simulink library "AEMS_Standard_Library"  (R2016b)
settings: Solver=ode45  StartTime=0.0  StopTime=10.0  RelTol=1e-3
undefined symbols (not defined in the file or in its folder): BkPY, carto, Cbx_extegr, Cbx_lpegrsys, Cbx_portegr, Cnx_bnk_nr_conf, Cnx_cyl_nr_conf, ConfigManagement, configuration_management, Cxx_dcm_io_tmr_end_xxxx, Cxx_dcm_rt_tmr_end, Cxx_DID_xxxx_IO_max, Cxx_DID_xxxx_IO_min, Cxx_egrhsofs, Cxx_vmaniegi, DEM_DEBOUNCE_FREEZE, DEM_DTR_CTL_INVISIBLE, DEM_DTR_CTL_NORMAL, Dem_DtrId2_XXX, Dem_DtrId3_XXX, Dem_DtrId4_XXX, Dem_DtrId5_XXX, Dem_DtrId6_XXX, Dem_DtrId7_XXX, Dem_DtrId8_XXX, Dem_DtrId9_XXX, Dem_DtrId_XXX, Dem_EnableConditionId2_XXX, Dem_EnableConditionId3_XXX, Dem_EnableConditionId4_XXX, Dem_EnableConditionId5_XXX, Dem_EnableConditionId6_XXX, Dem_EnableConditionId7_XXX, Dem_EnableConditionId8_XXX, Dem_EnableConditionId_XXX, Dem_EventId, Dem_EventId2_XXX, Dem_EventId3_XXX, Dem_EventId4_XXX, Dem_EventId5_XXX, Dem_EventId6_XXX, Dem_EventId7_XXX, Dem_EventId8_XXX, Dem_EventId9_XXX, Dem_EventId_Device_Faulttype, Dem_EventId_XXX, DEM_IUMPR_GENERAL_DENOMINATOR, DEM_OPCYC_IGNITION, Dem_RatioId2_XXX, Dem_RatioId3_XXX, Dem_RatioId4_XXX, Dem_RatioId5_XXX, Dem_RatioId6_XXX, Dem_RatioId7_XXX, Dem_RatioId8_XXX, Dem_RatioId_XXX, Dem_StorageConditionId2_XXX, Dem_StorageConditionId3_XXX, Dem_StorageConditionId4_XXX, Dem_StorageConditionId5_XXX ... (+65)
libraries: AEMS_Standard_Library x477, simulink x2
(part 33 of 39)

== system AEMS_Standard_Library/SUB/AEMS_DEM_SET_DTR_8DU/Dem_SetDTR_Call8 ==
  testresult8 : Inport  Interpolate=off
  lowerlimit8 : Inport  Port=2  Interpolate=off
  upperlimit8 : Inport  Port=3  Interpolate=off
  ctrl_flag8 : Inport  Port=4  Interpolate=off
  set_flag8 : EnablePort
      settings: AttributesFormatString=<states=%<StatesWhenEnabling>>
  AEMS_DEM_SETDTR8 : AEMS_Standard_Library/SUB/AEMS_DEM_SETDTR  Tag=[LIB]
      settings: AttributesFormatString=%<MaskType>
  Ctrlval_block1 : Constant  Value=DEM_DTR_CTL_NORMAL  OutDataTypeStr=uint8
  Ctrlval_block2 : Constant  Value=DEM_DTR_CTL_INVISIBLE  OutDataTypeStr=uint8
  DTRId_block8 : Constant  Value=Dem_DtrId8_XXX  OutDataTypeStr=uint16
  Data Type Conversion : DataTypeConversion  OutDataTypeStr=int32  SaturateOnIntegerOverflow=on
  Data Type Conversion1 : DataTypeConversion  OutDataTypeStr=int32  SaturateOnIntegerOverflow=on
  Data Type Conversion2 : DataTypeConversion  OutDataTypeStr=int32  SaturateOnIntegerOverflow=on
  Limitter22 : Saturate  UpperLimit=1  LowerLimit=0
      settings: AttributesFormatString=<limits=%<UpperLimit>/%<LowerLimit>>
  Limitter23 : Saturate  UpperLimit=1  LowerLimit=0
      settings: AttributesFormatString=<limits=%<UpperLimit>/%<LowerLimit>>
  Limitter24 : Saturate  UpperLimit=1  LowerLimit=0
      settings: AttributesFormatString=<limits=%<UpperLimit>/%<LowerLimit>>
  Sum : Sum  OutDataTypeStr=Inherit: Inherit via back propagation  SaturateOnIntegerOverflow=on  InputSameDT=on
  Sum1 : Sum  OutDataTypeStr=Inherit: Inherit via back propagation  SaturateOnIntegerOverflow=on  InputSameDT=on
  Sum2 : Sum  OutDataTypeStr=Inherit: Inherit via back propagation  SaturateOnIntegerOverflow=on  InputSameDT=on
  Switch : Switch  Criteria=u2 ~= 0  ZeroCross=off  InputSameDT=on
      settings: AttributesFormatString=Criteria=%<Criteria>
  offset1 : Constant  Value=0  OutDataTypeStr=uint16
  offset2 : Constant  Value=0  OutDataTypeStr=uint16
  offset3 : Constant  Value=0  OutDataTypeStr=uint16
  wires:
  Data Type Conversion2/1 -> AEMS_DEM_SETDTR8/4  "uplimit8"
  Data Type Conversion1/1 -> AEMS_DEM_SETDTR8/3  "lowlimit8"
  Data Type Conversion/1 -> AEMS_DEM_SETDTR8/2  "result8"
  DTRId_block8/1 -> AEMS_DEM_SETDTR8/1  "dtrid8"
  upperlimit8/1 -> Limitter24/1
  lowerlimit8/1 -> Limitter23/1
  testresult8/1 -> Limitter22/1
  Sum2/1 -> Data Type Conversion2/1
  Sum1/1 -> Data Type Conversion1/1
  Sum/1 -> Data Type Conversion/1
  Limitter24/1 -> Sum2/2
  offset3/1 -> Sum2/1
  Limitter23/1 -> Sum1/2
  offset2/1 -> Sum1/1
  Limitter22/1 -> Sum/2
  offset1/1 -> Sum/1
  Ctrlval_block1/1 -> Switch/1
  ctrl_flag8/1 -> Switch/2
  Ctrlval_block2/1 -> Switch/3
  Switch/1 -> AEMS_DEM_SETDTR8/5  "ctrlval8"

== system AEMS_Standard_Library/SUB/AEMS_DEM_SET_DTR_9DU/Dem_SetDTR_Call0 ==
  testresult0 : Inport  Interpolate=off
      settings: AttributesFormatString=<tsample=%<SampleTime>>
  lowerlimit0 : Inport  Port=2  Interpolate=off
      settings: AttributesFormatString=<tsample=%<SampleTime>>
  upperlimit0 : Inport  Port=3  Interpolate=off
      settings: AttributesFormatString=<tsample=%<SampleTime>>
  ctrl_flag0 : Inport  Port=4  Interpolate=off
      settings: AttributesFormatString=<tsample=%<SampleTime>>
  set_flag0 : EnablePort
      settings: AttributesFormatString=<states=%<StatesWhenEnabling>>
  AEMS_DEM_SETDTR : AEMS_Standard_Library/SUB/AEMS_DEM_SETDTR  Tag=[LIB]
      settings: AttributesFormatString=%<MaskType>
  Ctrlval_block1 : Constant  Value=DEM_DTR_CTL_NORMAL  OutDataTypeStr=uint8
  Ctrlval_block2 : Constant  Value=DEM_DTR_CTL_INVISIBLE  OutDataTypeStr=uint8
  DTRId_block0 : Constant  Value=Dem_DtrId_XXX  OutDataTypeStr=uint16
  Data Type Conversion : DataTypeConversion  OutDataTypeStr=int32  SaturateOnIntegerOverflow=on
  Data Type Conversion1 : DataTypeConversion  OutDataTypeStr=int32  SaturateOnIntegerOverflow=on
  Data Type Conversion2 : DataTypeConversion  OutDataTypeStr=int32  SaturateOnIntegerOverflow=on
  Limitter25 : Saturate  UpperLimit=1  LowerLimit=0
      settings: AttributesFormatString=<limits=%<UpperLimit>/%<LowerLimit>>
  Limitter26 : Saturate  UpperLimit=1  LowerLimit=0
      settings: AttributesFormatString=<limits=%<UpperLimit>/%<LowerLimit>>
  Limitter27 : Saturate  UpperLimit=1  LowerLimit=0
      settings: AttributesFormatString=<limits=%<UpperLimit>/%<LowerLimit>>
  Sum : Sum  SaturateOnIntegerOverflow=on  InputSameDT=on
  Sum1 : Sum  SaturateOnIntegerOverflow=on  InputSameDT=on
  Sum2 : Sum  SaturateOnIntegerOverflow=on  InputSameDT=on
  Switch : Switch  Threshold=0.5  ZeroCross=off  InputSameDT=on
  offset25 : Constant  Value=0  OutDataTypeStr=uint16
  offset26 : Constant  Value=0  OutDataTypeStr=uint16
  offset27 : Constant  Value=0  OutDataTypeStr=uint16
  wires:
  Ctrlval_block2/1 -> Switch/3
  ctrl_flag0/1 -> Switch/2
  Ctrlval_block1/1 -> Switch/1
  Switch/1 -> AEMS_DEM_SETDTR/5  "ctrlval0"
  offset25/1 -> Sum/1
  Limitter25/1 -> Sum/2
  offset26/1 -> Sum1/1
  Limitter26/1 -> Sum1/2
  offset27/1 -> Sum2/1
  Limitter27/1 -> Sum2/2
  Sum/1 -> Data Type Conversion/1
  Sum1/1 -> Data Type Conversion1/1
  Sum2/1 -> Data Type Conversion2/1
  testresult0/1 -> Limitter25/1
  lowerlimit0/1 -> Limitter26/1
  upperlimit0/1 -> Limitter27/1
  DTRId_block0/1 -> AEMS_DEM_SETDTR/1  "dtrid0"
  Data Type Conversion/1 -> AEMS_DEM_SETDTR/2  "result0"
  Data Type Conversion1/1 -> AEMS_DEM_SETDTR/3  "lowlimit0"
  Data Type Conversion2/1 -> AEMS_DEM_SETDTR/4  "uplimit0"

== system AEMS_Standard_Library/SUB/AEMS_DEM_SET_DTR_9DU/Dem_SetDTR_Call1 ==
  testresult1 : Inport  Interpolate=off
      settings: AttributesFormatString=<tsample=%<SampleTime>>
  lowerlimit1 : Inport  Port=2  Interpolate=off
      settings: AttributesFormatString=<tsample=%<SampleTime>>
  upperlimit1 : Inport  Port=3  Interpolate=off
      settings: AttributesFormatString=<tsample=%<SampleTime>>
  ctrl_flag1 : Inport  Port=4  Interpolate=off
      settings: AttributesFormatString=<tsample=%<SampleTime>>
  set_flag1 : EnablePort
      settings: AttributesFormatString=<states=%<StatesWhenEnabling>>
  AEMS_DEM_SETDTR : AEMS_Standard_Library/SUB/AEMS_DEM_SETDTR  Tag=[LIB]
      settings: AttributesFormatString=%<MaskType>
  Ctrlval_block1 : Constant  Value=DEM_DTR_CTL_NORMAL  OutDataTypeStr=uint8
  Ctrlval_block2 : Constant  Value=DEM_DTR_CTL_INVISIBLE  OutDataTypeStr=uint8
  DTRId_block1 : Constant  Value=Dem_DtrId2_XXX  OutDataTypeStr=uint16
  Data Type Conversion : DataTypeConversion  OutDataTypeStr=int32  SaturateOnIntegerOverflow=on
  Data Type Conversion1 : DataTypeConversion  OutDataTypeStr=int32  SaturateOnIntegerOverflow=on
  Data Type Conversion2 : DataTypeConversion  OutDataTypeStr=int32  SaturateOnIntegerOverflow=on
  Limitter1 : Saturate  UpperLimit=1  LowerLimit=0
      settings: AttributesFormatString=<limits=%<UpperLimit>/%<LowerLimit>>
  Limitter2 : Saturate  UpperLimit=1  LowerLimit=0
      settings: AttributesFormatString=<limits=%<UpperLimit>/%<LowerLimit>>
  Limitter3 : Saturate  UpperLimit=1  LowerLimit=0
      settings: AttributesFormatString=<limits=%<UpperLimit>/%<LowerLimit>>
  Sum : Sum  SaturateOnIntegerOverflow=on  InputSameDT=on
  Sum1 : Sum  SaturateOnIntegerOverflow=on  InputSameDT=on
  Sum2 : Sum  SaturateOnIntegerOverflow=on  InputSameDT=on
  Switch : Switch  Threshold=0.5  ZeroCross=off  InputSameDT=on
  offset1 : Constant  Value=0  OutDataTypeStr=uint16
  offset2 : Constant  Value=0  OutDataTypeStr=uint16
  offset3 : Constant  Value=0  OutDataTypeStr=uint16
  wires:
  Data Type Conversion2/1 -> AEMS_DEM_SETDTR/4  "uplimit1"
  Data Type Conversion1/1 -> AEMS_DEM_SETDTR/3  "lowlimit1"
  Data Type Conversion/1 -> AEMS_DEM_SETDTR/2  "result1"
  DTRId_block1/1 -> AEMS_DEM_SETDTR/1  "dtrid1"
  upperlimit1/1 -> Limitter3/1
  lowerlimit1/1 -> Limitter2/1
  testresult1/1 -> Limitter1/1
  Sum2/1 -> Data Type Conversion2/1
  Sum1/1 -> Data Type Conversion1/1
  Sum/1 -> Data Type Conversion/1
  Limitter3/1 -> Sum2/2
  offset3/1 -> Sum2/1
  Limitter2/1 -> Sum1/2
  offset2/1 -> Sum1/1
  Limitter1/1 -> Sum/2
  offset1/1 -> Sum/1
  Switch/1 -> AEMS_DEM_SETDTR/5  "ctrlval1"
  Ctrlval_block1/1 -> Switch/1
  ctrl_flag1/1 -> Switch/2
  Ctrlval_block2/1 -> Switch/3

== system AEMS_Standard_Library/SUB/AEMS_DEM_SET_DTR_9DU/Dem_SetDTR_Call2 ==
  testresult2 : Inport  Interpolate=off
      settings: AttributesFormatString=<tsample=%<SampleTime>>
  lowerlimit2 : Inport  Port=2  Interpolate=off
      settings: AttributesFormatString=<tsample=%<SampleTime>>
  upperlimit2 : Inport  Port=3  Interpolate=off
      settings: AttributesFormatString=<tsample=%<SampleTime>>
  ctrl_flag2 : Inport  Port=4  Interpolate=off
      settings: AttributesFormatString=<tsample=%<SampleTime>>
  set_flag2 : EnablePort
      settings: AttributesFormatString=<states=%<StatesWhenEnabling>>
  AEMS_DEM_SETDTR : AEMS_Standard_Library/SUB/AEMS_DEM_SETDTR  Tag=[LIB]
      settings: AttributesFormatString=%<MaskType>
  Ctrlval_block1 : Constant  Value=DEM_DTR_CTL_NORMAL  OutDataTypeStr=uint8
  Ctrlval_block2 : Constant  Value=DEM_DTR_CTL_INVISIBLE  OutDataTypeStr=uint8
  DTRId_block2 : Constant  Value=Dem_DtrId3_XXX  OutDataTypeStr=uint16
  Data Type Conversion : DataTypeConversion  OutDataTypeStr=int32  SaturateOnIntegerOverflow=on
  Data Type Conversion1 : DataTypeConversion  OutDataTypeStr=int32  SaturateOnIntegerOverflow=on
  Data Type Conversion2 : DataTypeConversion  OutDataTypeStr=int32  SaturateOnIntegerOverflow=on
  Limitter4 : Saturate  UpperLimit=1  LowerLimit=0
      settings: AttributesFormatString=<limits=%<UpperLimit>/%<LowerLimit>>
  Limitter5 : Saturate  UpperLimit=1  LowerLimit=0
      settings: AttributesFormatString=<limits=%<UpperLimit>/%<LowerLimit>>
  Limitter6 : Saturate  UpperLimit=1  LowerLimit=0
      settings: AttributesFormatString=<limits=%<UpperLimit>/%<LowerLimit>>
  Sum : Sum  SaturateOnIntegerOverflow=on  InputSameDT=on
  Sum1 : Sum  SaturateOnIntegerOverflow=on  InputSameDT=on
  Sum2 : Sum  SaturateOnIntegerOverflow=on  InputSameDT=on
  Switch : Switch  Threshold=0.5  ZeroCross=off  InputSameDT=on
  offset1 : Constant  Value=0  OutDataTypeStr=uint16
  offset2 : Constant  Value=0  OutDataTypeStr=uint16
  offset3 : Constant  Value=0  OutDataTypeStr=uint16
  wires:
  Data Type Conversion2/1 -> AEMS_DEM_SETDTR/4  "uplimit2"
  Data Type Conversion1/1 -> AEMS_DEM_SETDTR/3  "lowlimit2"
  Data Type Conversion/1 -> AEMS_DEM_SETDTR/2  "result2"
  DTRId_block2/1 -> AEMS_DEM_SETDTR/1  "dtrid2"
  upperlimit2/1 -> Limitter6/1
  lowerlimit2/1 -> Limitter5/1
  testresult2/1 -> Limitter4/1
  Sum2/1 -> Data Type Conversion2/1
  Sum1/1 -> Data Type Conversion1/1
  Sum/1 -> Data Type Conversion/1
  Limitter6/1 -> Sum2/2
  offset3/1 -> Sum2/1
  Limitter5/1 -> Sum1/2
  offset2/1 -> Sum1/1
  Limitter4/1 -> Sum/2
  offset1/1 -> Sum/1
  Ctrlval_block1/1 -> Switch/1
  ctrl_flag2/1 -> Switch/2
  Ctrlval_block2/1 -> Switch/3
  Switch/1 -> AEMS_DEM_SETDTR/5  "ctrlval2"

== system AEMS_Standard_Library/SUB/AEMS_DEM_SET_DTR_9DU/Dem_SetDTR_Call3 ==
  testresult3 : Inport  Interpolate=off
      settings: AttributesFormatString=<tsample=%<SampleTime>>
  lowerlimit3 : Inport  Port=2  Interpolate=off
      settings: AttributesFormatString=<tsample=%<SampleTime>>
  upperlimit3 : Inport  Port=3  Interpolate=off
      settings: AttributesFormatString=<tsample=%<SampleTime>>
  ctrl_flag3 : Inport  Port=4  Interpolate=off
      settings: AttributesFormatString=<tsample=%<SampleTime>>
  set_flag3 : EnablePort
      settings: AttributesFormatString=<states=%<StatesWhenEnabling>>
  AEMS_DEM_SETDTR : AEMS_Standard_Library/SUB/AEMS_DEM_SETDTR  Tag=[LIB]
      settings: AttributesFormatString=%<MaskType>
  Ctrlval_block1 : Constant  Value=DEM_DTR_CTL_NORMAL  OutDataTypeStr=uint8
  Ctrlval_block2 : Constant  Value=DEM_DTR_CTL_INVISIBLE  OutDataTypeStr=uint8
  DTRId_block3 : Constant  Value=Dem_DtrId4_XXX  OutDataTypeStr=uint16
  Data Type Conversion : DataTypeConversion  OutDataTypeStr=int32  SaturateOnIntegerOverflow=on
  Data Type Conversion1 : DataTypeConversion  OutDataTypeStr=int32  SaturateOnIntegerOverflow=on
  Data Type Conversion2 : DataTypeConversion  OutDataTypeStr=int32  SaturateOnIntegerOverflow=on
  Limitter7 : Saturate  UpperLimit=1  LowerLimit=0
      settings: AttributesFormatString=<limits=%<UpperLimit>/%<LowerLimit>>
  Limitter8 : Saturate  UpperLimit=1  LowerLimit=0
      settings: AttributesFormatString=<limits=%<UpperLimit>/%<LowerLimit>>
  Limitter9 : Saturate  UpperLimit=1  LowerLimit=0
      settings: AttributesFormatString=<limits=%<UpperLimit>/%<LowerLimit>>
  Sum : Sum  SaturateOnIntegerOverflow=on  InputSameDT=on
  Sum1 : Sum  SaturateOnIntegerOverflow=on  InputSameDT=on
  Sum2 : Sum  SaturateOnIntegerOverflow=on  InputSameDT=on
  Switch : Switch  Threshold=0.5  ZeroCross=off  InputSameDT=on
  offset1 : Constant  Value=0  OutDataTypeStr=uint16
  offset2 : Constant  Value=0  OutDataTypeStr=uint16
  offset3 : Constant  Value=0  OutDataTypeStr=uint16
  wires:
  Data Type Conversion2/1 -> AEMS_DEM_SETDTR/4  "uplimit3"
  Data Type Conversion1/1 -> AEMS_DEM_SETDTR/3  "lowlimit3"
  Data Type Conversion/1 -> AEMS_DEM_SETDTR/2  "result3"
  DTRId_block3/1 -> AEMS_DEM_SETDTR/1  "dtrid3"
  upperlimit3/1 -> Limitter9/1
  lowerlimit3/1 -> Limitter8/1
  testresult3/1 -> Limitter7/1
  Sum2/1 -> Data Type Conversion2/1
  Sum1/1 -> Data Type Conversion1/1
  Sum/1 -> Data Type Conversion/1
  Limitter9/1 -> Sum2/2
  offset3/1 -> Sum2/1
  Limitter8/1 -> Sum1/2
  offset2/1 -> Sum1/1
  Limitter7/1 -> Sum/2
  offset1/1 -> Sum/1
  Ctrlval_block1/1 -> Switch/1
  ctrl_flag3/1 -> Switch/2
  Ctrlval_block2/1 -> Switch/3
  Switch/1 -> AEMS_DEM_SETDTR/5  "ctrlval3"

== system AEMS_Standard_Library/SUB/AEMS_DEM_SET_DTR_9DU/Dem_SetDTR_Call4 ==
  testresult4 : Inport  Interpolate=off
      settings: AttributesFormatString=<tsample=%<SampleTime>>
  lowerlimit4 : Inport  Port=2  Interpolate=off
      settings: AttributesFormatString=<tsample=%<SampleTime>>
  upperlimit4 : Inport  Port=3  Interpolate=off
      settings: AttributesFormatString=<tsample=%<SampleTime>>
  ctrl_flag4 : Inport  Port=4  Interpolate=off
      settings: AttributesFormatString=<tsample=%<SampleTime>>
  set_flag4 : EnablePort
      settings: AttributesFormatString=<states=%<StatesWhenEnabling>>
  AEMS_DEM_SETDTR : AEMS_Standard_Library/SUB/AEMS_DEM_SETDTR  Tag=[LIB]
      settings: AttributesFormatString=%<MaskType>
  Ctrlval_block1 : Constant  Value=DEM_DTR_CTL_NORMAL  OutDataTypeStr=uint8
  Ctrlval_block2 : Constant  Value=DEM_DTR_CTL_INVISIBLE  OutDataTypeStr=uint8
  DTRId_block4 : Constant  Value=Dem_DtrId5_XXX  OutDataTypeStr=uint16
  Data Type Conversion : DataTypeConversion  OutDataTypeStr=int32  SaturateOnIntegerOverflow=on
  Data Type Conversion1 : DataTypeConversion  OutDataTypeStr=int32  SaturateOnIntegerOverflow=on
  Data Type Conversion2 : DataTypeConversion  OutDataTypeStr=int32  SaturateOnIntegerOverflow=on
  Limitter10 : Saturate  UpperLimit=1  LowerLimit=0
      settings: AttributesFormatString=<limits=%<UpperLimit>/%<LowerLimit>>
  Limitter11 : Saturate  UpperLimit=1  LowerLimit=0
      settings: AttributesFormatString=<limits=%<UpperLimit>/%<LowerLimit>>
  Limitter12 : Saturate  UpperLimit=1  LowerLimit=0
      settings: AttributesFormatString=<limits=%<UpperLimit>/%<LowerLimit>>
  Sum : Sum  SaturateOnIntegerOverflow=on  InputSameDT=on
  Sum1 : Sum  SaturateOnIntegerOverflow=on  InputSameDT=on
  Sum2 : Sum  SaturateOnIntegerOverflow=on  InputSameDT=on
  Switch : Switch  Threshold=0.5  ZeroCross=off  InputSameDT=on
  offset1 : Constant  Value=0  OutDataTypeStr=uint16
  offset2 : Constant  Value=0  OutDataTypeStr=uint16
  offset3 : Constant  Value=0  OutDataTypeStr=uint16
  wires:
  Data Type Conversion2/1 -> AEMS_DEM_SETDTR/4  "uplimit4"
  Data Type Conversion1/1 -> AEMS_DEM_SETDTR/3  "lowlimit4"
  Data Type Conversion/1 -> AEMS_DEM_SETDTR/2  "result4"
  DTRId_block4/1 -> AEMS_DEM_SETDTR/1  "dtrid4"
  upperlimit4/1 -> Limitter12/1
  lowerlimit4/1 -> Limitter11/1
  testresult4/1 -> Limitter10/1
  Sum2/1 -> Data Type Conversion2/1
  Sum1/1 -> Data Type Conversion1/1
  Sum/1 -> Data Type Conversion/1
  Limitter12/1 -> Sum2/2
  offset3/1 -> Sum2/1
  Limitter11/1 -> Sum1/2
  offset2/1 -> Sum1/1
  Limitter10/1 -> Sum/2
  offset1/1 -> Sum/1
  Ctrlval_block1/1 -> Switch/1
  ctrl_flag4/1 -> Switch/2
  Ctrlval_block2/1 -> Switch/3
  Switch/1 -> AEMS_DEM_SETDTR/5  "ctrlval4"

== system AEMS_Standard_Library/SUB/AEMS_DEM_SET_DTR_9DU/Dem_SetDTR_Call5 ==
  testresult5 : Inport  Interpolate=off
      settings: AttributesFormatString=<tsample=%<SampleTime>>
  lowerlimit5 : Inport  Port=2  Interpolate=off
      settings: AttributesFormatString=<tsample=%<SampleTime>>
  upperlimit5 : Inport  Port=3  Interpolate=off
      settings: AttributesFormatString=<tsample=%<SampleTime>>
  ctrl_flag5 : Inport  Port=4  Interpolate=off
      settings: AttributesFormatString=<tsample=%<SampleTime>>
  set_flag5 : EnablePort
      settings: AttributesFormatString=<states=%<StatesWhenEnabling>>
  AEMS_DEM_SETDTR : AEMS_Standard_Library/SUB/AEMS_DEM_SETDTR  Tag=[LIB]
      settings: AttributesFormatString=%<MaskType>
  Ctrlval_block1 : Constant  Value=DEM_DTR_CTL_NORMAL  OutDataTypeStr=uint8
  Ctrlval_block2 : Constant  Value=DEM_DTR_CTL_INVISIBLE  OutDataTypeStr=uint8
  DTRId_block5 : Constant  Value=Dem_DtrId6_XXX  OutDataTypeStr=uint16
  Data Type Conversion : DataTypeConversion  OutDataTypeStr=int32  SaturateOnIntegerOverflow=on
  Data Type Conversion1 : DataTypeConversion  OutDataTypeStr=int32  SaturateOnIntegerOverflow=on
  Data Type Conversion2 : DataTypeConversion  OutDataTypeStr=int32  SaturateOnIntegerOverflow=on
  Limitter13 : Saturate  UpperLimit=1  LowerLimit=0
      settings: AttributesFormatString=<limits=%<UpperLimit>/%<LowerLimit>>
  Limitter14 : Saturate  UpperLimit=1  LowerLimit=0
      settings: AttributesFormatString=<limits=%<UpperLimit>/%<LowerLimit>>
  Limitter15 : Saturate  UpperLimit=1  LowerLimit=0
      settings: AttributesFormatString=<limits=%<UpperLimit>/%<LowerLimit>>
  Sum : Sum  SaturateOnIntegerOverflow=on  InputSameDT=on
  Sum1 : Sum  SaturateOnIntegerOverflow=on  InputSameDT=on
  Sum2 : Sum  SaturateOnIntegerOverflow=on  InputSameDT=on
  Switch : Switch  Threshold=0.5  ZeroCross=off  InputSameDT=on
  offset1 : Constant  Value=0  OutDataTypeStr=uint16
  offset2 : Constant  Value=0  OutDataTypeStr=uint16
  offset3 : Constant  Value=0  OutDataTypeStr=uint16
  wires:
  Data Type Conversion2/1 -> AEMS_DEM_SETDTR/4  "uplimit5"
  Data Type Conversion1/1 -> AEMS_DEM_SETDTR/3  "lowlimit5"
  Data Type Conversion/1 -> AEMS_DEM_SETDTR/2  "result5"
  DTRId_block5/1 -> AEMS_DEM_SETDTR/1  "dtrid5"
  upperlimit5/1 -> Limitter15/1
  lowerlimit5/1 -> Limitter14/1
  testresult5/1 -> Limitter13/1
  Sum2/1 -> Data Type Conversion2/1
  Sum1/1 -> Data Type Conversion1/1
  Sum/1 -> Data Type Conversion/1
  Limitter15/1 -> Sum2/2
  offset3/1 -> Sum2/1
  Limitter14/1 -> Sum1/2
  offset2/1 -> Sum1/1
  Limitter13/1 -> Sum/2
  offset1/1 -> Sum/1
  Ctrlval_block1/1 -> Switch/1
  ctrl_flag5/1 -> Switch/2
  Ctrlval_block2/1 -> Switch/3
  Switch/1 -> AEMS_DEM_SETDTR/5  "ctrlval5"

== system AEMS_Standard_Library/SUB/AEMS_DEM_SET_DTR_9DU/Dem_SetDTR_Call6 ==
  testresult6 : Inport  Interpolate=off
      settings: AttributesFormatString=<tsample=%<SampleTime>>
  lowerlimit6 : Inport  Port=2  Interpolate=off
      settings: AttributesFormatString=<tsample=%<SampleTime>>
  upperlimit6 : Inport  Port=3  Interpolate=off
      settings: AttributesFormatString=<tsample=%<SampleTime>>
  ctrl_flag6 : Inport  Port=4  Interpolate=off
      settings: AttributesFormatString=<tsample=%<SampleTime>>
  set_flag6 : EnablePort
      settings: AttributesFormatString=<states=%<StatesWhenEnabling>>
  AEMS_DEM_SETDTR : AEMS_Standard_Library/SUB/AEMS_DEM_SETDTR  Tag=[LIB]
      settings: AttributesFormatString=%<MaskType>
  Ctrlval_block1 : Constant  Value=DEM_DTR_CTL_NORMAL  OutDataTypeStr=uint8
  Ctrlval_block2 : Constant  Value=DEM_DTR_CTL_INVISIBLE  OutDataTypeStr=uint8
  DTRId_block6 : Constant  Value=Dem_DtrId7_XXX  OutDataTypeStr=uint16
  Data Type Conversion : DataTypeConversion  OutDataTypeStr=int32  SaturateOnIntegerOverflow=on
  Data Type Conversion1 : DataTypeConversion  OutDataTypeStr=int32  SaturateOnIntegerOverflow=on
  Data Type Conversion2 : DataTypeConversion  OutDataTypeStr=int32  SaturateOnIntegerOverflow=on
  Limitter16 : Saturate  UpperLimit=1  LowerLimit=0
      settings: AttributesFormatString=<limits=%<UpperLimit>/%<LowerLimit>>
  Limitter17 : Saturate  UpperLimit=1  LowerLimit=0
      settings: AttributesFormatString=<limits=%<UpperLimit>/%<LowerLimit>>
  Limitter18 : Saturate  UpperLimit=1  LowerLimit=0
      settings: AttributesFormatString=<limits=%<UpperLimit>/%<LowerLimit>>
  Sum : Sum  SaturateOnIntegerOverflow=on  InputSameDT=on
  Sum1 : Sum  SaturateOnIntegerOverflow=on  InputSameDT=on
  Sum2 : Sum  SaturateOnIntegerOverflow=on  InputSameDT=on
  Switch : Switch  Threshold=0.5  ZeroCross=off  InputSameDT=on
  offset1 : Constant  Value=0  OutDataTypeStr=uint16
  offset2 : Constant  Value=0  OutDataTypeStr=uint16
  offset3 : Constant  Value=0  OutDataTypeStr=uint16
  wires:
  Data Type Conversion2/1 -> AEMS_DEM_SETDTR/4  "uplimit6"
  Data Type Conversion1/1 -> AEMS_DEM_SETDTR/3  "lowlimit6"
  Data Type Conversion/1 -> AEMS_DEM_SETDTR/2  "result6"
  DTRId_block6/1 -> AEMS_DEM_SETDTR/1  "dtrid6"
  upperlimit6/1 -> Limitter18/1
  lowerlimit6/1 -> Limitter17/1
  testresult6/1 -> Limitter16/1
  Sum2/1 -> Data Type Conversion2/1
  Sum1/1 -> Data Type Conversion1/1
  Sum/1 -> Data Type Conversion/1
  Limitter18/1 -> Sum2/2
  offset3/1 -> Sum2/1
  Limitter17/1 -> Sum1/2
  offset2/1 -> Sum1/1
  Limitter16/1 -> Sum/2
  offset1/1 -> Sum/1
  Ctrlval_block1/1 -> Switch/1
  ctrl_flag6/1 -> Switch/2
  Ctrlval_block2/1 -> Switch/3
  Switch/1 -> AEMS_DEM_SETDTR/5  "ctrlval6"

== system AEMS_Standard_Library/SUB/AEMS_DEM_SET_DTR_9DU/Dem_SetDTR_Call7 ==
  testresult7 : Inport  Interpolate=off
      settings: AttributesFormatString=<tsample=%<SampleTime>>
  lowerlimit7 : Inport  Port=2  Interpolate=off
      settings: AttributesFormatString=<tsample=%<SampleTime>>
  upperlimit7 : Inport  Port=3  Interpolate=off
      settings: AttributesFormatString=<tsample=%<SampleTime>>
  ctrl_flag7 : Inport  Port=4  Interpolate=off
      settings: AttributesFormatString=<tsample=%<SampleTime>>
  set_flag7 : EnablePort
      settings: AttributesFormatString=<states=%<StatesWhenEnabling>>
  AEMS_DEM_SETDTR : AEMS_Standard_Library/SUB/AEMS_DEM_SETDTR  Tag=[LIB]
      settings: AttributesFormatString=%<MaskType>
  Ctrlval_block1 : Constant  Value=DEM_DTR_CTL_NORMAL  OutDataTypeStr=uint8
  Ctrlval_block2 : Constant  Value=DEM_DTR_CTL_INVISIBLE  OutDataTypeStr=uint8
  DTRId_block7 : Constant  Value=Dem_DtrId8_XXX  OutDataTypeStr=uint16
  Data Type Conversion : DataTypeConversion  OutDataTypeStr=int32  SaturateOnIntegerOverflow=on
  Data Type Conversion1 : DataTypeConversion  OutDataTypeStr=int32  SaturateOnIntegerOverflow=on
  Data Type Conversion2 : DataTypeConversion  OutDataTypeStr=int32  SaturateOnIntegerOverflow=on
  Limitter19 : Saturate  UpperLimit=1  LowerLimit=0
      settings: AttributesFormatString=<limits=%<UpperLimit>/%<LowerLimit>>
  Limitter20 : Saturate  UpperLimit=1  LowerLimit=0
      settings: AttributesFormatString=<limits=%<UpperLimit>/%<LowerLimit>>
  Limitter21 : Saturate  UpperLimit=1  LowerLimit=0
      settings: AttributesFormatString=<limits=%<UpperLimit>/%<LowerLimit>>
  Sum : Sum  SaturateOnIntegerOverflow=on  InputSameDT=on
  Sum1 : Sum  SaturateOnIntegerOverflow=on  InputSameDT=on
  Sum2 : Sum  SaturateOnIntegerOverflow=on  InputSameDT=on
  Switch : Switch  Threshold=0.5  ZeroCross=off  InputSameDT=on
  offset1 : Constant  Value=0  OutDataTypeStr=uint16
  offset2 : Constant  Value=0  OutDataTypeStr=uint16
  offset3 : Constant  Value=0  OutDataTypeStr=uint16
  wires:
  Data Type Conversion2/1 -> AEMS_DEM_SETDTR/4  "uplimit7"
  Data Type Conversion1/1 -> AEMS_DEM_SETDTR/3  "lowlimit7"
  Data Type Conversion/1 -> AEMS_DEM_SETDTR/2  "result7"
  DTRId_block7/1 -> AEMS_DEM_SETDTR/1  "dtrid7"
  upperlimit7/1 -> Limitter21/1
  lowerlimit7/1 -> Limitter20/1
  testresult7/1 -> Limitter19/1
  Sum2/1 -> Data Type Conversion2/1
  Sum1/1 -> Data Type Conversion1/1
  Sum/1 -> Data Type Conversion/1
  Limitter21/1 -> Sum2/2
  offset3/1 -> Sum2/1
  Limitter20/1 -> Sum1/2
  offset2/1 -> Sum1/1
  Limitter19/1 -> Sum/2
  offset1/1 -> Sum/1
  Ctrlval_block1/1 -> Switch/1
  ctrl_flag7/1 -> Switch/2
  Ctrlval_block2/1 -> Switch/3
  Switch/1 -> AEMS_DEM_SETDTR/5  "ctrlval7"

== system AEMS_Standard_Library/SUB/AEMS_DEM_SET_DTR_9DU/Dem_SetDTR_Call8 ==
  testresult8 : Inport  Interpolate=off
      settings: AttributesFormatString=<tsample=%<SampleTime>>
  lowerlimit8 : Inport  Port=2  Interpolate=off
      settings: AttributesFormatString=<tsample=%<SampleTime>>
  upperlimit8 : Inport  Port=3  Interpolate=off
      settings: AttributesFormatString=<tsample=%<SampleTime>>
  ctrl_flag8 : Inport  Port=4  Interpolate=off
      settings: AttributesFormatString=<tsample=%<SampleTime>>
  set_flag8 : EnablePort
      settings: AttributesFormatString=<states=%<StatesWhenEnabling>>
  AEMS_DEM_SETDTR : AEMS_Standard_Library/SUB/AEMS_DEM_SETDTR  Tag=[LIB]
      settings: AttributesFormatString=%<MaskType>
  Ctrlval_block1 : Constant  Value=DEM_DTR_CTL_NORMAL  OutDataTypeStr=uint8
  Ctrlval_block2 : Constant  Value=DEM_DTR_CTL_INVISIBLE  OutDataTypeStr=uint8
  DTRId_block8 : Constant  Value=Dem_DtrId9_XXX  OutDataTypeStr=uint16
  Data Type Conversion : DataTypeConversion  OutDataTypeStr=int32  SaturateOnIntegerOverflow=on
  Data Type Conversion1 : DataTypeConversion  OutDataTypeStr=int32  SaturateOnIntegerOverflow=on
  Data Type Conversion2 : DataTypeConversion  OutDataTypeStr=int32  SaturateOnIntegerOverflow=on
  Limitter22 : Saturate  UpperLimit=1  LowerLimit=0
      settings: AttributesFormatString=<limits=%<UpperLimit>/%<LowerLimit>>
  Limitter23 : Saturate  UpperLimit=1  LowerLimit=0
      settings: AttributesFormatString=<limits=%<UpperLimit>/%<LowerLimit>>
  Limitter24 : Saturate  UpperLimit=1  LowerLimit=0
      settings: AttributesFormatString=<limits=%<UpperLimit>/%<LowerLimit>>
  Sum : Sum  SaturateOnIntegerOverflow=on  InputSameDT=on
  Sum1 : Sum  SaturateOnIntegerOverflow=on  InputSameDT=on
  Sum2 : Sum  SaturateOnIntegerOverflow=on  InputSameDT=on
  Switch : Switch  Threshold=0.5  ZeroCross=off  InputSameDT=on
  offset1 : Constant  Value=0  OutDataTypeStr=uint16
  offset2 : Constant  Value=0  OutDataTypeStr=uint16
  offset3 : Constant  Value=0  OutDataTypeStr=uint16
  wires:
  Data Type Conversion2/1 -> AEMS_DEM_SETDTR/4  "uplimit8"
  Data Type Conversion1/1 -> AEMS_DEM_SETDTR/3  "lowlimit8"
  Data Type Conversion/1 -> AEMS_DEM_SETDTR/2  "result8"
  DTRId_block8/1 -> AEMS_DEM_SETDTR/1  "dtrid8"
  upperlimit8/1 -> Limitter24/1
  lowerlimit8/1 -> Limitter23/1
  testresult8/1 -> Limitter22/1
  Sum2/1 -> Data Type Conversion2/1
  Sum1/1 -> Data Type Conversion1/1
  Sum/1 -> Data Type Conversion/1
  Limitter24/1 -> Sum2/2
  offset3/1 -> Sum2/1
  Limitter23/1 -> Sum1/2
  offset2/1 -> Sum1/1
  Limitter22/1 -> Sum/2
  offset1/1 -> Sum/1
  Ctrlval_block1/1 -> Switch/1
  ctrl_flag8/1 -> Switch/2
  Ctrlval_block2/1 -> Switch/3
  Switch/1 -> AEMS_DEM_SETDTR/5  "ctrlval8"

== system AEMS_Standard_Library/SUB/AEMS_DEM_SET_EVENT_AVL_1D/DEM_SET_EVENT_AVL_E ==
  trigger_job_1st : EnablePort
      settings: AttributesFormatString=<states=%<StatesWhenEnabling>>
  AEMS_DEM_SETEVENTAVAILABLE : AEMS_Standard_Library/SUB/AEMS_DEM_SETEVENTAVAILABLE
      settings: AttributesFormatString=%<MaskType>
  Diagnosis_SW : Constant  Value=Diag_ROMFLAG  OutDataTypeStr=boolean
  EventId_block : Constant  Value=EventID  OutDataTypeStr=uint16
  dgnsw : Outport  InitialOutput=0
      settings: AttributesFormatString=<initial=%<InitialOutput>>\n<whendisabled=%<outputwhendisabled>>
  wires:
  Diagnosis_SW/1 -> AEMS_DEM_SETEVENTAVAILABLE/2, dgnsw/1  "dgnsw"
  EventId_block/1 -> AEMS_DEM_SETEVENTAVAILABLE/1

== system AEMS_Standard_Library/SUB/AEMS_DEM_SET_EVENT_AVL_2D/DEM_SET_EVENT_AVL_E ==
  trigger_job_1st : EnablePort
      settings: AttributesFormatString=<states=%<StatesWhenEnabling>>
  AEMS_DEM_SETEVENTAVAILABLE1 : AEMS_Standard_Library/SUB/AEMS_DEM_SETEVENTAVAILABLE  Tag=[LIB]
      settings: AttributesFormatString=%<MaskType>
  AEMS_DEM_SETEVENTAVAILABLE2 : AEMS_Standard_Library/SUB/AEMS_DEM_SETEVENTAVAILABLE  Tag=[LIB]
      settings: AttributesFormatString=%<MaskType>
  Constant1 : Constant  OutDataTypeStr=uint8
  Constant2 : Constant  Value=[1 0]  OutDataTypeStr=boolean
  Constant3 : Constant  Value=[1 1]  OutDataTypeStr=boolean
  Demux : Demux  Outputs=2
  Diagnosis_SW : Constant  Value=mfXXX  OutDataTypeStr=boolean
  EventId_block1 : Constant  Value=Dem_EventId_XXX  OutDataTypeStr=uint16
  EventId_block2 : Constant  Value=Dem_EventId2_XXX  OutDataTypeStr=uint16
  LogicalOperator : Logic  OutDataTypeStr=boolean
  RelationalOperator : RelationalOperator  Operator===  OutDataTypeStr=boolean  RndMeth=Nearest  InputSameDT=on
  Switch : Switch  Criteria=u2 ~= 0  SaturateOnIntegerOverflow=on  InputSameDT=on
      settings: AttributesFormatString=Criteria=%<Criteria>
  index_parameter : Constant  Value=Cnx_bnk_nr_conf
  dgnsw : Outport  InitialOutput=0
      settings: AttributesFormatString=<initial=%<InitialOutput>>\n<whendisabled=%<outputwhendisabled>>
  wires:
  Demux/2 -> AEMS_DEM_SETEVENTAVAILABLE2/2
  Demux/1 -> AEMS_DEM_SETEVENTAVAILABLE1/2
  EventId_block2/1 -> AEMS_DEM_SETEVENTAVAILABLE2/1
  EventId_block1/1 -> AEMS_DEM_SETEVENTAVAILABLE1/1
  Constant3/1 -> Switch/3
  Constant2/1 -> Switch/1
  Constant1/1 -> RelationalOperator/1
  RelationalOperator/1 -> Switch/2
  Diagnosis_SW/1 -> LogicalOperator/2
  Switch/1 -> LogicalOperator/1
  LogicalOperator/1 -> Demux/1, dgnsw/1  "dgnsw"
  index_parameter/1 -> RelationalOperator/2

== system AEMS_Standard_Library/SUB/AEMS_DEM_SET_EVENT_AVL_8D/DEM_SET_EVENT_AVL_E ==
  trigger_job_1st : EnablePort
      settings: AttributesFormatString=<states=%<StatesWhenEnabling>>
  AEMS_DEM_SETEVENTAVAILABLE{1..8} (8 alike) : AEMS_Standard_Library/SUB/AEMS_DEM_SETEVENTAVAILABLE  Tag=[LIB]
      settings: AttributesFormatString=%<MaskType>
  Constant1 : Constant  Value=3  OutDataTypeStr=uint8
  Constant2 : Constant  Value=[1 1 1 0 0 0 0 0]  OutDataTypeStr=boolean
  Constant3 : Constant  Value=[1 1 1 1 0 0 0 0]  OutDataTypeStr=boolean
  Constant4 : Constant  Value=4  OutDataTypeStr=uint8
  Constant5 : Constant  Value=[1 1 1 1 1 1 0 0]  OutDataTypeStr=boolean
  Constant6 : Constant  Value=6  OutDataTypeStr=uint8
  Constant7 : Constant  Value=[1 1 1 1 1 1 1 1]  OutDataTypeStr=boolean
  Demux : Demux  Outputs=8
  Diagnosis_SW : Constant  Value=mfXXX  OutDataTypeStr=boolean
  EventId_block1 : Constant  Value=Dem_EventId_XXX  OutDataTypeStr=uint16
  EventId_block2 : Constant  Value=Dem_EventId2_XXX  OutDataTypeStr=uint16
  EventId_block3 : Constant  Value=Dem_EventId3_XXX  OutDataTypeStr=uint16
  EventId_block4 : Constant  Value=Dem_EventId4_XXX  OutDataTypeStr=uint16
  EventId_block5 : Constant  Value=Dem_EventId5_XXX  OutDataTypeStr=uint16
  EventId_block6 : Constant  Value=Dem_EventId6_XXX  OutDataTypeStr=uint16
  EventId_block7 : Constant  Value=Dem_EventId7_XXX  OutDataTypeStr=uint16
  EventId_block8 : Constant  Value=Dem_EventId8_XXX  OutDataTypeStr=uint16
  LogicalOperator : Logic  OutDataTypeStr=boolean
  RelationalOperator : RelationalOperator  Operator===  OutDataTypeStr=boolean  RndMeth=Nearest  InputSameDT=on
  RelationalOperator1 : RelationalOperator  Operator===  OutDataTypeStr=boolean  RndMeth=Nearest  InputSameDT=on
  RelationalOperator2 : RelationalOperator  Operator===  OutDataTypeStr=boolean  RndMeth=Nearest  InputSameDT=on
  Switch : Switch  Criteria=u2 ~= 0  SaturateOnIntegerOverflow=on  InputSameDT=on
      settings: AttributesFormatString=Criteria=%<Criteria>
  Switch1 : Switch  Criteria=u2 ~= 0  SaturateOnIntegerOverflow=on  InputSameDT=on
      settings: AttributesFormatString=Criteria=%<Criteria>
  Switch2 : Switch  Criteria=u2 ~= 0  SaturateOnIntegerOverflow=on  InputSameDT=on
      settings: AttributesFormatString=Criteria=%<Criteria>
  index_parameter : Constant  Value=Cnx_cyl_nr_conf
  dgnsw : Outport  InitialOutput=0
      settings: AttributesFormatString=<initial=%<InitialOutput>>\n<whendisabled=%<OutputWhenDisabled>>
  wires:
  index_parameter/1 -> RelationalOperator2/2, RelationalOperator1/2, RelationalOperator/2
  Constant7/1 -> Switch2/3  "cyl8"
  RelationalOperator2/1 -> Switch2/2
  Constant6/1 -> RelationalOperator2/1
  Constant5/1 -> Switch2/1  "cyl6"
  Switch2/1 -> Switch1/3
  RelationalOperator1/1 -> Switch1/2
  Constant4/1 -> RelationalOperator1/1
  Switch1/1 -> Switch/3
  EventId_block2/1 -> AEMS_DEM_SETEVENTAVAILABLE2/1
  EventId_block1/1 -> AEMS_DEM_SETEVENTAVAILABLE1/1
  EventId_block3/1 -> AEMS_DEM_SETEVENTAVAILABLE3/1
  EventId_block4/1 -> AEMS_DEM_SETEVENTAVAILABLE4/1
  EventId_block6/1 -> AEMS_DEM_SETEVENTAVAILABLE6/1
  EventId_block7/1 -> AEMS_DEM_SETEVENTAVAILABLE7/1
  EventId_block8/1 -> AEMS_DEM_SETEVENTAVAILABLE8/1
  Demux/1 -> AEMS_DEM_SETEVENTAVAILABLE1/2
  Demux/2 -> AEMS_DEM_SETEVENTAVAILABLE2/2
  Demux/3 -> AEMS_DEM_SETEVENTAVAILABLE3/2
  Demux/4 -> AEMS_DEM_SETEVENTAVAILABLE4/2
  EventId_block5/1 -> AEMS_DEM_SETEVENTAVAILABLE5/1
  Demux/5 -> AEMS_DEM_SETEVENTAVAILABLE5/2
  Demux/6 -> AEMS_DEM_SETEVENTAVAILABLE6/2
  Demux/7 -> AEMS_DEM_SETEVENTAVAILABLE7/2
  Demux/8 -> AEMS_DEM_SETEVENTAVAILABLE8/2
  Constant3/1 -> Switch1/1  "cyl4"
  Constant2/1 -> Switch/1  "cyl3"
  Constant1/1 -> RelationalOperator/1
  RelationalOperator/1 -> Switch/2
  Diagnosis_SW/1 -> LogicalOperator/1
  Switch/1 -> LogicalOperator/2
  LogicalOperator/1 -> dgnsw/1, Demux/1  "dgnsw"

== system AEMS_Standard_Library/SUB/AEMS_DEM_SET_EVENT_AVL_9D/DEM_SET_EVENT_AVL_E ==
  trigger_job_1st : EnablePort
      settings: AttributesFormatString=<states=%<StatesWhenEnabling>>
  AEMS_DEM_SETEVENTAVAILABLE{1..9} (9 alike) : AEMS_Standard_Library/SUB/AEMS_DEM_SETEVENTAVAILABLE  Tag=[LIB]
      settings: AttributesFormatString=%<MaskType>
  Constant1 : Constant  Value=3  OutDataTypeStr=uint8
  Constant2 : Constant  Value=[1 1 1 1 0 0 0 0 0]  OutDataTypeStr=boolean
  Constant3 : Constant  Value=[1 1 1 1 1 0 0 0 0]  OutDataTypeStr=boolean
  Constant4 : Constant  Value=4  OutDataTypeStr=uint8
  Constant5 : Constant  Value=[1 1 1 1 1 1 1 0 0]  OutDataTypeStr=boolean
  Constant6 : Constant  Value=6  OutDataTypeStr=uint8
  Constant7 : Constant  Value=[1 1 1 1 1 1 1 1 1]  OutDataTypeStr=boolean
  Demux : Demux  Outputs=9
  Diagnosis_SW : Constant  Value=mfXXX  OutDataTypeStr=boolean
  EventId_block0 : Constant  Value=Dem_EventId_XXX  OutDataTypeStr=uint16
  EventId_block1 : Constant  Value=Dem_EventId2_XXX  OutDataTypeStr=uint16
  EventId_block2 : Constant  Value=Dem_EventId3_XXX  OutDataTypeStr=uint16
  EventId_block3 : Constant  Value=Dem_EventId4_XXX  OutDataTypeStr=uint16
  EventId_block4 : Constant  Value=Dem_EventId5_XXX  OutDataTypeStr=uint16
  EventId_block5 : Constant  Value=Dem_EventId6_XXX  OutDataTypeStr=uint16
  EventId_block6 : Constant  Value=Dem_EventId7_XXX  OutDataTypeStr=uint16
  EventId_block7 : Constant  Value=Dem_EventId8_XXX  OutDataTypeStr=uint16
  EventId_block8 : Constant  Value=Dem_EventId9_XXX  OutDataTypeStr=uint16
  LogicalOperator : Logic  OutDataTypeStr=boolean
  RelationalOperator : RelationalOperator  Operator===  OutDataTypeStr=boolean  RndMeth=Nearest  InputSameDT=on
  RelationalOperator1 : RelationalOperator  Operator===  OutDataTypeStr=boolean  RndMeth=Nearest  InputSameDT=on
  RelationalOperator2 : RelationalOperator  Operator===  OutDataTypeStr=boolean  RndMeth=Nearest  InputSameDT=on
  Switch : Switch  Threshold=0.5  SaturateOnIntegerOverflow=on  InputSameDT=on
  Switch1 : Switch  Threshold=0.5  SaturateOnIntegerOverflow=on  InputSameDT=on
  Switch2 : Switch  Threshold=0.5  SaturateOnIntegerOverflow=on  InputSameDT=on
  index_parameter : Constant  Value=Cnx_cyl_nr_conf
  dgnsw : Outport  InitialOutput=0
      settings: AttributesFormatString=<initial=%<InitialOutput>>\n<WhenDisabled=%<OutputWhenDisabled>>
  wires:
  Demux/9 -> AEMS_DEM_SETEVENTAVAILABLE9/2
  Demux/8 -> AEMS_DEM_SETEVENTAVAILABLE8/2
  Demux/7 -> AEMS_DEM_SETEVENTAVAILABLE7/2
  Demux/6 -> AEMS_DEM_SETEVENTAVAILABLE6/2
  Demux/5 -> AEMS_DEM_SETEVENTAVAILABLE5/2
  Demux/4 -> AEMS_DEM_SETEVENTAVAILABLE4/2
  Demux/3 -> AEMS_DEM_SETEVENTAVAILABLE3/2
  Demux/2 -> AEMS_DEM_SETEVENTAVAILABLE2/2
  Demux/1 -> AEMS_DEM_SETEVENTAVAILABLE1/2
  EventId_block0/1 -> AEMS_DEM_SETEVENTAVAILABLE1/1
  LogicalOperator/1 -> Demux/1, dgnsw/1  "dgnsw"
  Switch/1 -> LogicalOperator/2
  Diagnosis_SW/1 -> LogicalOperator/1
  RelationalOperator/1 -> Switch/2
  Constant1/1 -> RelationalOperator/1
  Constant2/1 -> Switch/1  "cyl3"
  Constant3/1 -> Switch1/1  "cyl4"
  EventId_block5/1 -> AEMS_DEM_SETEVENTAVAILABLE6/1
  EventId_block8/1 -> AEMS_DEM_SETEVENTAVAILABLE9/1
  EventId_block7/1 -> AEMS_DEM_SETEVENTAVAILABLE8/1
  EventId_block6/1 -> AEMS_DEM_SETEVENTAVAILABLE7/1
  EventId_block4/1 -> AEMS_DEM_SETEVENTAVAILABLE5/1
  EventId_block3/1 -> AEMS_DEM_SETEVENTAVAILABLE4/1
  EventId_block1/1 -> AEMS_DEM_SETEVENTAVAILABLE2/1
  EventId_block2/1 -> AEMS_DEM_SETEVENTAVAILABLE3/1
  Switch1/1 -> Switch/3
  Constant4/1 -> RelationalOperator1/1
  RelationalOperator1/1 -> Switch1/2
  Switch2/1 -> Switch1/3
  Constant5/1 -> Switch2/1  "cyl6"
  Constant6/1 -> RelationalOperator2/1
  RelationalOperator2/1 -> Switch2/2
  Constant7/1 -> Switch2/3  "cyl8"
  index_parameter/1 -> RelationalOperator/2, RelationalOperator1/2, RelationalOperator2/2

== system AEMS_Standard_Library/SUB/AEMS_DEM_SET_EVENT_DSBL_1D/Dem_SetEventDisabled_Call ==
  set_flag : EnablePort
      settings: AttributesFormatString=<states=%<StatesWhenEnabling>>
  AEMS_DEM_SETEVENTDISABLED : AEMS_Standard_Library/SUB/AEMS_DEM_SETEVENTDISABLED  Tag=[LIB]
      settings: AttributesFormatString=%<MaskType>
  EventId_block : Constant  Value=Dem_EventId_XXX  OutDataTypeStr=uint16
  wires:
  EventId_block/1 -> AEMS_DEM_SETEVENTDISABLED/1  "eventid"

== system AEMS_Standard_Library/SUB/AEMS_DEM_SET_EVENT_DSBL_2D/Dem_SetEventDisabled_Call1 ==
  set_flag1 : EnablePort
      settings: AttributesFormatString=<states=%<StatesWhenEnabling>>
  AEMS_DEM_SETEVENTDISABLED1 : AEMS_Standard_Library/SUB/AEMS_DEM_SETEVENTDISABLED  Tag=[LIB]
      settings: AttributesFormatString=%<MaskType>
  EventId_block1 : Constant  Value=Dem_EventId_XXX  OutDataTypeStr=uint16
  wires:
  EventId_block1/1 -> AEMS_DEM_SETEVENTDISABLED1/1  "eventid1"

== system AEMS_Standard_Library/SUB/AEMS_DEM_SET_EVENT_DSBL_2D/Dem_SetEventDisabled_Call2 ==
  set_flag2 : EnablePort
      settings: AttributesFormatString=<states=%<StatesWhenEnabling>>
  AEMS_DEM_SETEVENTDISABLED2 : AEMS_Standard_Library/SUB/AEMS_DEM_SETEVENTDISABLED  Tag=[LIB]
      settings: AttributesFormatString=%<MaskType>
  EventId_block2 : Constant  Value=Dem_EventId2_XXX  OutDataTypeStr=uint16
  wires:
  EventId_block2/1 -> AEMS_DEM_SETEVENTDISABLED2/1  "eventid2"

== system AEMS_Standard_Library/SUB/AEMS_DEM_SET_EVENT_DSBL_8D/Dem_SetEventDisabled_Call1 ==
  set_flag1 : EnablePort
      settings: AttributesFormatString=<states=%<StatesWhenEnabling>>
  AEMS_DEM_SETEVENTDISABLED1 : AEMS_Standard_Library/SUB/AEMS_DEM_SETEVENTDISABLED  Tag=[LIB]
      settings: AttributesFormatString=%<MaskType>
  EventId_block1 : Constant  Value=Dem_EventId_XXX  OutDataTypeStr=uint16
  wires:
  EventId_block1/1 -> AEMS_DEM_SETEVENTDISABLED1/1  "eventid1"

== system AEMS_Standard_Library/SUB/AEMS_DEM_SET_EVENT_DSBL_8D/Dem_SetEventDisabled_Call2 ==
  set_flag2 : EnablePort
      settings: AttributesFormatString=<states=%<StatesWhenEnabling>>
  AEMS_DEM_SETEVENTDISABLED2 : AEMS_Standard_Library/SUB/AEMS_DEM_SETEVENTDISABLED  Tag=[LIB]
      settings: AttributesFormatString=%<MaskType>
  EventId_block2 : Constant  Value=Dem_EventId2_XXX  OutDataTypeStr=uint16
  wires:
  EventId_block2/1 -> AEMS_DEM_SETEVENTDISABLED2/1  "eventid2"

== system AEMS_Standard_Library/SUB/AEMS_DEM_SET_EVENT_DSBL_8D/Dem_SetEventDisabled_Call3 ==
  set_flag3 : EnablePort
      settings: AttributesFormatString=<states=%<StatesWhenEnabling>>
  AEMS_DEM_SETEVENTDISABLED3 : AEMS_Standard_Library/SUB/AEMS_DEM_SETEVENTDISABLED  Tag=[LIB]
      settings: AttributesFormatString=%<MaskType>
  EventId_block3 : Constant  Value=Dem_EventId3_XXX  OutDataTypeStr=uint16
  wires:
  EventId_block3/1 -> AEMS_DEM_SETEVENTDISABLED3/1  "eventid3"

== system AEMS_Standard_Library/SUB/AEMS_DEM_SET_EVENT_DSBL_8D/Dem_SetEventDisabled_Call4 ==
  set_flag4 : EnablePort
      settings: AttributesFormatString=<states=%<StatesWhenEnabling>>
  AEMS_DEM_SETEVENTDISABLED4 : AEMS_Standard_Library/SUB/AEMS_DEM_SETEVENTDISABLED  Tag=[LIB]
      settings: AttributesFormatString=%<MaskType>
  EventId_block4 : Constant  Value=Dem_EventId4_XXX  OutDataTypeStr=uint16
  wires:
  EventId_block4/1 -> AEMS_DEM_SETEVENTDISABLED4/1  "eventid4"

== system AEMS_Standard_Library/SUB/AEMS_DEM_SET_EVENT_DSBL_8D/Dem_SetEventDisabled_Call5 ==
  set_flag5 : EnablePort
      settings: AttributesFormatString=<states=%<StatesWhenEnabling>>
  AEMS_DEM_SETEVENTDISABLED5 : AEMS_Standard_Library/SUB/AEMS_DEM_SETEVENTDISABLED  Tag=[LIB]
      settings: AttributesFormatString=%<MaskType>
  EventId_block5 : Constant  Value=Dem_EventId5_XXX  OutDataTypeStr=uint16
  wires:
  EventId_block5/1 -> AEMS_DEM_SETEVENTDISABLED5/1  "eventid5"

== system AEMS_Standard_Library/SUB/AEMS_DEM_SET_EVENT_DSBL_8D/Dem_SetEventDisabled_Call6 ==
  set_flag6 : EnablePort
      settings: AttributesFormatString=<states=%<StatesWhenEnabling>>
  AEMS_DEM_SETEVENTDISABLED6 : AEMS_Standard_Library/SUB/AEMS_DEM_SETEVENTDISABLED  Tag=[LIB]
      settings: AttributesFormatString=%<MaskType>
  EventId_block6 : Constant  Value=Dem_EventId6_XXX  OutDataTypeStr=uint16
  wires:
  EventId_block6/1 -> AEMS_DEM_SETEVENTDISABLED6/1  "eventid6"

== system AEMS_Standard_Library/SUB/AEMS_DEM_SET_EVENT_DSBL_8D/Dem_SetEventDisabled_Call7 ==
  set_flag7 : EnablePort
      settings: AttributesFormatString=<states=%<StatesWhenEnabling>>
  AEMS_DEM_SETEVENTDISABLED7 : AEMS_Standard_Library/SUB/AEMS_DEM_SETEVENTDISABLED  Tag=[LIB]
      settings: AttributesFormatString=%<MaskType>
  EventId_block7 : Constant  Value=Dem_EventId7_XXX  OutDataTypeStr=uint16
  wires:
  EventId_block7/1 -> AEMS_DEM_SETEVENTDISABLED7/1  "eventid7"

== system AEMS_Standard_Library/SUB/AEMS_DEM_SET_EVENT_DSBL_8D/Dem_SetEventDisabled_Call8 ==
  set_flag8 : EnablePort
      settings: AttributesFormatString=<states=%<StatesWhenEnabling>>
  AEMS_DEM_SETEVENTDISABLED8 : AEMS_Standard_Library/SUB/AEMS_DEM_SETEVENTDISABLED  Tag=[LIB]
      settings: AttributesFormatString=%<MaskType>
  EventId_block8 : Constant  Value=Dem_EventId8_XXX  OutDataTypeStr=uint16
  wires:
  EventId_block8/1 -> AEMS_DEM_SETEVENTDISABLED8/1  "eventid8"

== system AEMS_Standard_Library/SUB/AEMS_DEM_SET_EVENT_DSBL_9D/Dem_SetEventDisabled_Call0 ==
  set_flag0 : EnablePort
      settings: AttributesFormatString=<states=%<StatesWhenEnabling>>
  AEMS_DEM_SETEVENTDISABLED : AEMS_Standard_Library/SUB/AEMS_DEM_SETEVENTDISABLED  Tag=[LIB]
      settings: AttributesFormatString=%<MaskType>
  EventId_block0 : Constant  Value=Dem_EventId_XXX  OutDataTypeStr=uint16
  wires:
  EventId_block0/1 -> AEMS_DEM_SETEVENTDISABLED/1  "eventid1"

== system AEMS_Standard_Library/SUB/AEMS_DEM_SET_EVENT_DSBL_9D/Dem_SetEventDisabled_Call1 ==
  set_flag1 : EnablePort
      settings: AttributesFormatString=<states=%<StatesWhenEnabling>>
  AEMS_DEM_SETEVENTDISABLED : AEMS_Standard_Library/SUB/AEMS_DEM_SETEVENTDISABLED  Tag=[LIB]
      settings: AttributesFormatString=%<MaskType>
  EventId_block1 : Constant  Value=Dem_EventId2_XXX  OutDataTypeStr=uint16
  wires:
  EventId_block1/1 -> AEMS_DEM_SETEVENTDISABLED/1  "eventid1"

== system AEMS_Standard_Library/SUB/AEMS_DEM_SET_EVENT_DSBL_9D/Dem_SetEventDisabled_Call2 ==
  set_flag2 : EnablePort
      settings: AttributesFormatString=<states=%<StatesWhenEnabling>>
  AEMS_DEM_SETEVENTDISABLED : AEMS_Standard_Library/SUB/AEMS_DEM_SETEVENTDISABLED  Tag=[LIB]
      settings: AttributesFormatString=%<MaskType>
  EventId_block2 : Constant  Value=Dem_EventId3_XXX  OutDataTypeStr=uint16
  wires:
  EventId_block2/1 -> AEMS_DEM_SETEVENTDISABLED/1  "eventid2"

== system AEMS_Standard_Library/SUB/AEMS_DEM_SET_EVENT_DSBL_9D/Dem_SetEventDisabled_Call3 ==
  set_flag3 : EnablePort
      settings: AttributesFormatString=<states=%<StatesWhenEnabling>>
  AEMS_DEM_SETEVENTDISABLED : AEMS_Standard_Library/SUB/AEMS_DEM_SETEVENTDISABLED  Tag=[LIB]
      settings: AttributesFormatString=%<MaskType>
  EventId_block3 : Constant  Value=Dem_EventId4_XXX  OutDataTypeStr=uint16
  wires:
  EventId_block3/1 -> AEMS_DEM_SETEVENTDISABLED/1  "eventid3"

== system AEMS_Standard_Library/SUB/AEMS_DEM_SET_EVENT_DSBL_9D/Dem_SetEventDisabled_Call4 ==
  set_flag4 : EnablePort
      settings: AttributesFormatString=<states=%<StatesWhenEnabling>>
  AEMS_DEM_SETEVENTDISABLED : AEMS_Standard_Library/SUB/AEMS_DEM_SETEVENTDISABLED  Tag=[LIB]
      settings: AttributesFormatString=%<MaskType>
  EventId_block4 : Constant  Value=Dem_EventId5_XXX  OutDataTypeStr=uint16
  wires:
  EventId_block4/1 -> AEMS_DEM_SETEVENTDISABLED/1  "eventid4"

== system AEMS_Standard_Library/SUB/AEMS_DEM_SET_EVENT_DSBL_9D/Dem_SetEventDisabled_Call5 ==
  set_flag5 : EnablePort
      settings: AttributesFormatString=<states=%<StatesWhenEnabling>>
  AEMS_DEM_SETEVENTDISABLED : AEMS_Standard_Library/SUB/AEMS_DEM_SETEVENTDISABLED  Tag=[LIB]
      settings: AttributesFormatString=%<MaskType>
  EventId_block5 : Constant  Value=Dem_EventId6_XXX  OutDataTypeStr=uint16
  wires:
  EventId_block5/1 -> AEMS_DEM_SETEVENTDISABLED/1  "eventid5"

== system AEMS_Standard_Library/SUB/AEMS_DEM_SET_EVENT_DSBL_9D/Dem_SetEventDisabled_Call6 ==
  set_flag6 : EnablePort
      settings: AttributesFormatString=<states=%<StatesWhenEnabling>>
  AEMS_DEM_SETEVENTDISABLED : AEMS_Standard_Library/SUB/AEMS_DEM_SETEVENTDISABLED  Tag=[LIB]
      settings: AttributesFormatString=%<MaskType>
  EventId_block6 : Constant  Value=Dem_EventId7_XXX  OutDataTypeStr=uint16
  wires:
  EventId_block6/1 -> AEMS_DEM_SETEVENTDISABLED/1  "eventid6"

== system AEMS_Standard_Library/SUB/AEMS_DEM_SET_EVENT_DSBL_9D/Dem_SetEventDisabled_Call7 ==
  set_flag7 : EnablePort
      settings: AttributesFormatString=<states=%<StatesWhenEnabling>>
  AEMS_DEM_SETEVENTDISABLED : AEMS_Standard_Library/SUB/AEMS_DEM_SETEVENTDISABLED  Tag=[LIB]
      settings: AttributesFormatString=%<MaskType>
  EventId_block7 : Constant  Value=Dem_EventId8_XXX  OutDataTypeStr=uint16
  wires:
  EventId_block7/1 -> AEMS_DEM_SETEVENTDISABLED/1  "eventid7"

== system AEMS_Standard_Library/SUB/AEMS_DEM_SET_EVENT_DSBL_9D/Dem_SetEventDisabled_Call8 ==
  set_flag8 : EnablePort
      settings: AttributesFormatString=<states=%<StatesWhenEnabling>>
  AEMS_DEM_SETEVENTDISABLED : AEMS_Standard_Library/SUB/AEMS_DEM_SETEVENTDISABLED  Tag=[LIB]
      settings: AttributesFormatString=%<MaskType>
  EventId_block8 : Constant  Value=Dem_EventId9_XXX  OutDataTypeStr=uint16
  wires:
  EventId_block8/1 -> AEMS_DEM_SETEVENTDISABLED/1  "eventid8"

== system AEMS_Standard_Library/SUB/AEMS_DEM_SET_EVENT_STS_1D/Dem_SetEventStatus_Call ==
  dem_event_status_failed : Inport
  trigger_job_1st : EnablePort
      settings: AttributesFormatString=<states=%<StatesWhenEnabling>>
  AEMS_DEM_SETEVENTSTATUS : AEMS_Standard_Library/SUB/AEMS_DEM_SETEVENTSTATUS
      settings: AttributesFormatString=%<MaskType>
  EventId_block : Constant  Value=Dem_EventId_XXX  OutDataTypeStr=uint16
  wires:
  EventId_block/1 -> AEMS_DEM_SETEVENTSTATUS/1
  dem_event_status_failed/1 -> AEMS_DEM_SETEVENTSTATUS/2

== system AEMS_Standard_Library/SUB/AEMS_DEM_SET_EVENT_STS_2D/Dem_SetEventStatus_Call1 ==
  dem_event_status_failed1 : Inport
  trigger_job_1st1 : EnablePort
      settings: AttributesFormatString=<states=%<StatesWhenEnabling>>
  AEMS_DEM_SETEVENTSTATUS1 : AEMS_Standard_Library/SUB/AEMS_DEM_SETEVENTSTATUS  Tag=[LIB]
      settings: AttributesFormatString=%<MaskType>
  EventId_block1 : Constant  Value=Dem_EventId_XXX  OutDataTypeStr=uint16
  wires:
  dem_event_status_failed1/1 -> AEMS_DEM_SETEVENTSTATUS1/2
  EventId_block1/1 -> AEMS_DEM_SETEVENTSTATUS1/1
